simulink model "LR_Traject_Sim_compatible"  (R2017b)
settings: Solver=ode4  StartTime=0  StopTime=100  FixedStep=0.05  RelTol=1e-7
model workspace (MAT data in the model file):
  MCOS : class17 (value not decoded)
values from neighbouring files (symbols this model uses):
  Vull = 0.15    [TestBlowdownModel.m]    (also in runsim.m)
undefined symbols (not defined in the file or in its folder): avionics, CEAinterp, Conditions, Eng, Prop, Roc
libraries: simulink x1
(part 2 of 2)

== matlab function LR_Traject_Sim_compatible/MATLAB Function4 ==
  data: Xvelo input; CurrentAngle output; Yvelo input; rail_length input; VehicleVelo output; h input; launchangle input
function [CurrentAngle, VehicleVelo]  = CurrentAngle(Xvelo,Yvelo, rail_length, h, launchangle)

%This function's main purpose is to calculate current vehicle angle without
%using two simulink math blocks vs one function block.

%Pretty cool huh?

CurrentAngle = atan(Xvelo/Yvelo);
VehicleVelo = sqrt(Xvelo^2+Yvelo^2);

if h < rail_length
    CurrentAngle = launchangle;
end

== matlab function LR_Traject_Sim_compatible/Avionics Modelling/Total Pressure Transducer/MATLAB Function ==
  data: Pinf input; Ptotal output; rho input; M input
function Ptotal = fcn(Pinf, rho, M)
% Returns the total pressure, selecting an isentropic, or
% Rayleigh formula as appropriate
% Isentropic works just as well as incompressible for our purposes

y = 1.4;

if M > 1
    Ptotal = Pinf * ((((y + 1)^2 * M^2)/(4 * y * M^2 - 2 * (y - 1)))^(y/(y - 1))) * ((1 - y + 2 * y * M^2)/(y + 1));
else
    Ptotal = Pinf * (1 + ((y - 1) * M^2 / 2))^(y / (y - 1));
end
end

== matlab function LR_Traject_Sim_compatible/Avionics Modelling/MATLAB Function1 ==
  data: timestep input; vel input; lastheight input; height output
function height = fcn(timestep, vel, lastheight)

height = lastheight + timestep * vel;
end

== matlab function LR_Traject_Sim_compatible/Avionics Modelling/Predictor ==
  data: timestep input; time input; projected_apogee output; vel input; height input; est_cd input; est_A input; est_mass input; enabled input
function projected_apogee = fcn(timestep, time, vel, height, est_cd, est_A, est_mass, enabled)
if (enabled == 1)
    max_time = 100; %In case something goes wrong it doesn't go into an infinite loop
    
    %cd = 0.433;
    %A = 0.0190106696733447;
    %mass = 32.5516;
    
    cd = est_cd;
    A = est_A;
    mass = est_mass;
    
    while(true)
        lastheight = height;
        time = time + timestep;
        
        p = getStandardPressure(height);
        rho = p/(287.058*(getStandardTemperature(getGeopotential(height/1000))));
        
        accel = -9.81 - ((1/2)*rho*A*cd*vel^2)/mass;
        vel = vel + accel*timestep;
        height = height + vel*timestep;
        
        if(lastheight > height || time > max_time); break; end
    end
end
projected_apogee = height;
end

% stuff below this stolen from wikipedia
function pressure = getStandardPressure( altitude)

altitude = altitude / 1000.0;
geopot_height = getGeopotential(altitude);

t = getStandardTemperature(geopot_height);

pressure = 0;
if (geopot_height <= 11)
    pressure = 101325 * (288.15 / t)^( -5.255877);
elseif (geopot_height <= 20)
    pressure = 22632.06 * exp(-0.1577 * (geopot_height - 11));
elseif (geopot_height <= 32)
    pressure = 5474.889 * (216.65 / t)^( 34.16319);
elseif (geopot_height <= 47)
    pressure = 868.0187 * (228.65 / t)^( 12.2011);
elseif (geopot_height <= 51)
    pressure = 110.9063 * exp(-0.1262 * (geopot_height - 47));
elseif (geopot_height <= 71)
    pressure = 66.93887 * (270.65 / t)^( -12.2011);
elseif (geopot_height <= 84.85)
    pressure = 3.956420 * (214.65 / t)^( -17.0816);
end

end

function temperature = getStandardTemperature(geopot_height)

temperature = 273.15;
if (geopot_height <= 11)
    temperature = 288.15 - (6.5 * geopot_height);
elseif (geopot_height <= 20)
    temperature = 216.65;
elseif (geopot_height <= 32)
    temperature = 196.65 + geopot_height;
elseif (geopot_height <= 47)
    temperature = 228.65 + 2.8 * (geopot_height - 32);
elseif (geopot_height <= 51)
    temperature = 270.65;
elseif (geopot_height <= 71)
    temperature = 270.65 - 2.8 * (geopot_height - 51);
elseif (geopot_height <= 84.85)
    temperature = 214.65 - 2 * (geopot_height - 71); 
end

end

function geopot = getGeopotential(altitude_km)

EARTH_RADIUS = 6356.766;

geopot = EARTH_RADIUS * altitude_km / (EARTH_RADIUS + altitude_km);
end
